simulink model "DC_mOTOR_VERSION2"  (R2022a)
settings: Solver=VariableStepAuto  StartTime=0.0  StopTime=10.0  RelTol=1e-3
settings Model: Creator=DELL  LastModifiedBy=DELL

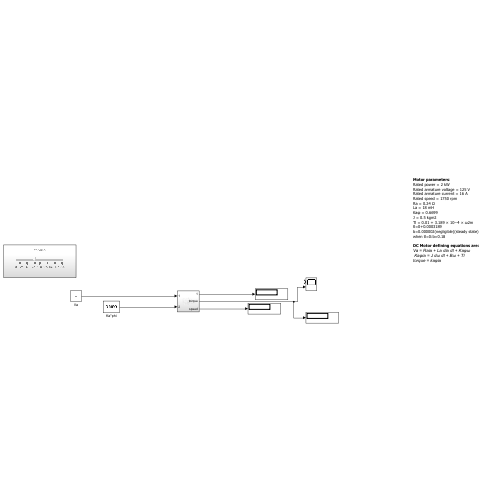
[thumbnail: Simulink's stored preview of the top-level diagram]
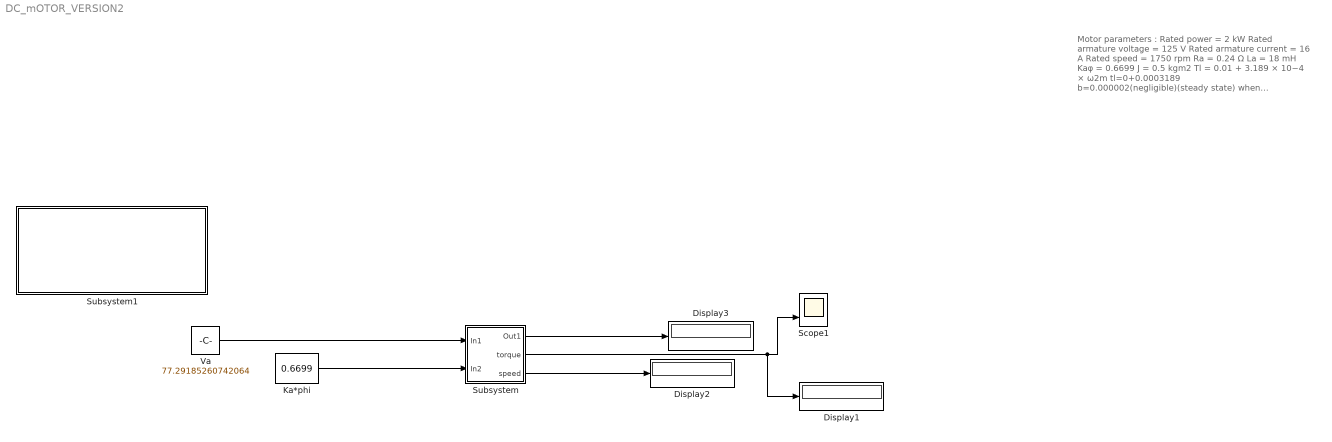
== system DC_mOTOR_VERSION2 ==
  note: Motor parameters :
      | Rated power = 2 kW
      | Rated armature voltage = 125 V
      | Rated armature current = 16 A
      | Rated speed = 1750 rpm
      | Ra = 0.24 Ω
      | La = 18 mH
      | Kaφ = 0.6699
      | J = 0.5 kgm2
      | Tl = 0.01 + 3.189 × 10−4 × ω2m
      | tl=0+0.0003189
      | b=0.000002(negligible)(steady state)
      | when tl=0:b=0.18
      |
      | DC Motor defining equations are:
      | Va = Raia + La dia dt + Kaφω
      | Kaφia = J dω dt + Bω + Tl
      | torque = kaφia
  Display1 : Display
  Display2 : Display
  Display3 : Display
  Ka*phi : Constant  Value=0.6699
  Scope1 : Scope  NumInputPorts=2
  Subsystem : Subsystem
  Subsystem1 : Subsystem
  Va : Constant  Value=77.29185260742064
  wires:
  Subsystem/3(speed) -> Display2/1
  Va/1 -> Subsystem/1(In1)
  Subsystem/1(Out1) -> Display3/1
  Subsystem/2(torque) -> Scope1/2, Display1/1
  Ka*phi/1 -> Subsystem/2(In2)

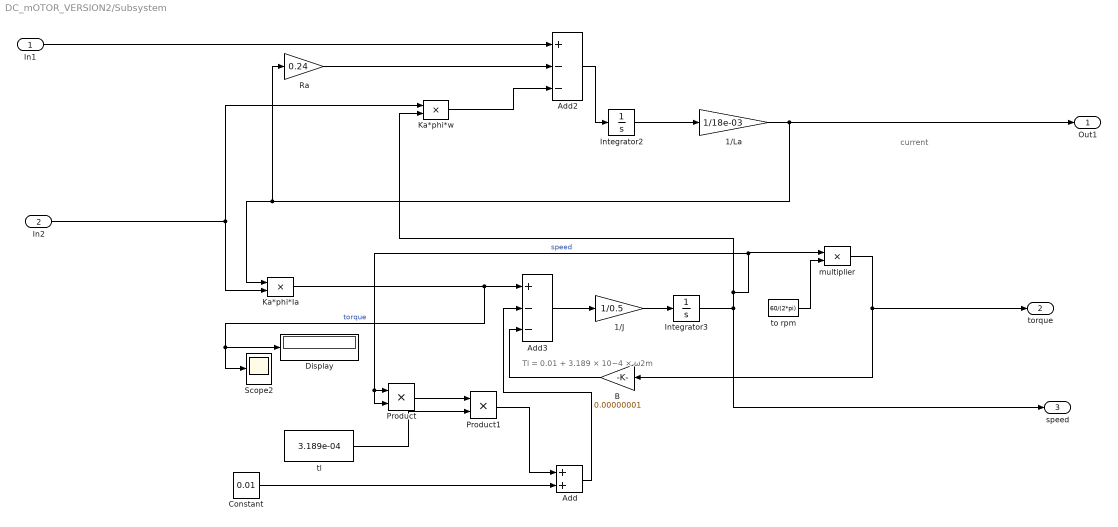
== system DC_mOTOR_VERSION2/Subsystem ==
  note: current
  note: Tl = 0.01 + 3.189 × 10−4 × ω2m
  In1 : Inport
  In2 : Inport  Port=2
  1/J : Gain  Gain=1/0.5
  1/La : Gain  Gain=1/18e-03
  Add : Sum
  Add2 : Sum  Inputs=+--
  Add3 : Sum  Inputs=+--
  B : Gain  Gain=0.00000001
  Constant : Constant  Value=0.01
  Display : Display
  Integrator2 : Integrator
  Integrator3 : Integrator
  Ka*phi*Ia : Product
  Ka*phi*w : Product
  Product : Product
  Product1 : Product
  Ra : Gain  Gain=0.24
  Scope2 : Scope
  multiplier : Product
  tl : Constant  Value=3.189e-04
  to rpm : Constant  Value=60/(2*pi)
  Out1 : Outport
  torque : Outport  Port=2
  speed : Outport  Port=3
  wires:
  Add2/1 -> Integrator2/1
  B/1 -> Add3/3
  Integrator3/1 -> speed/1, Ka*phi*w/2, Product/2, Product/1, multiplier/1  "speed"
  Ka*phi*w/1 -> Add2/3
  Add3/1 -> 1/J/1
  1/J/1 -> Integrator3/1
  tl/1 -> Product1/2
  Ra/1 -> Add2/2
  Ka*phi*Ia/1 -> Display/1, Scope2/1, Add3/1  "torque"
  Product1/1 -> Add/1
  In2/1 -> Ka*phi*Ia/2, Ka*phi*w/1
  multiplier/1 -> torque/1, B/1
  In1/1 -> Add2/1
  to rpm/1 -> multiplier/2
  1/La/1 -> Ka*phi*Ia/1, Ra/1, Out1/1
  Constant/1 -> Add/2
  Integrator2/1 -> 1/La/1
  Add/1 -> Add3/2
  Product/1 -> Product1/1

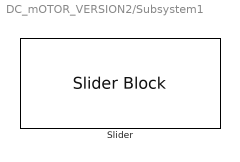
== system DC_mOTOR_VERSION2/Subsystem1 ==
  Slider : SliderBlock  ScaleMax=200
